simulink model "quy_dao_nghiem_so_2022"  (R2023b)
settings: Solver=VariableStepAuto  StartTime=0.0  StopTime=30000  MaxStep=20000.0  RelTol=1e-3
values from neighbouring files (symbols this model uses):
  A = 1    [doi_tuong.m]    (also in quy_dao_nghiem_so.m; tong_hop_truc_tiep.m)
  den = [1, a1, a2]    [quy_dao_nghiem_so.m]
  K1 = (alpha * l1_bar) / (2 * sqrt(delta_h))    [quy_dao_nghiem_so.m]
  K2 = (alpha * l2_bar) / (2 * sqrt(h2_bar))    [quy_dao_nghiem_so.m]
  K3 = alpha * sqrt(delta_h)    [quy_dao_nghiem_so.m]
  K4 = alpha * sqrt(h2_bar)    [quy_dao_nghiem_so.m]
libraries: simulink x2, slpidlib x2
settings Model: Creator=PC  LastModifiedBy=Moderator
settings SolverCC: ZeroCrossAlgorithm=Adaptive
settings DebuggingCC: IgnoredZcDiagnostic=none
settings RTWCC: GPUComputeCapability=5.0

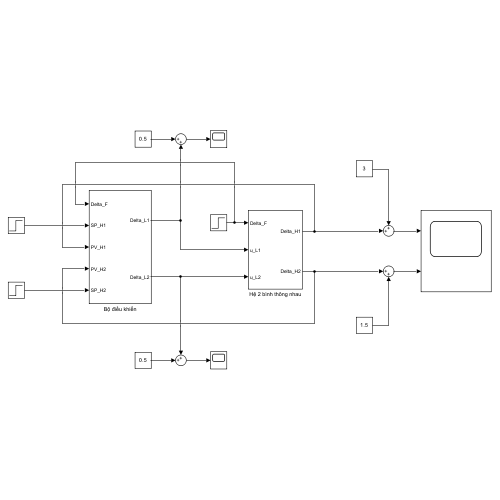
[thumbnail: Simulink's stored preview of the top-level diagram]
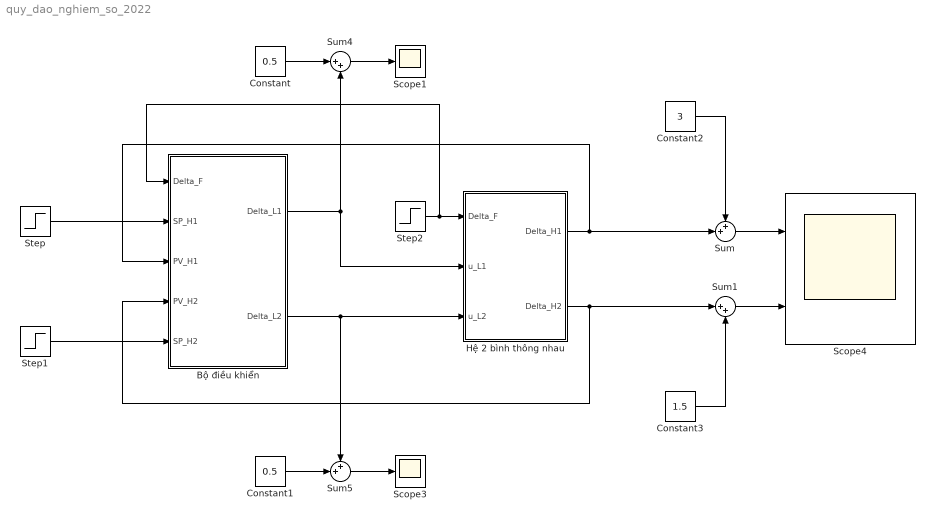
== system quy_dao_nghiem_so_2022 ==
  Bộ điều khiển : Subsystem
  Constant : Constant  Value=0.5
  Constant1 : Constant  Value=0.5
  Constant2 : Constant  Value=3
  Constant3 : Constant  Value=1.5
  Hệ 2 bình thông nhau : Subsystem
  Scope1 : Scope
  Scope3 : Scope
  Scope4 : Scope  NumInputPorts=2
  Step : Step  Time=20000  After=0.1  SampleTime=0
  Step1 : Step  Time=10000  After=0.1  SampleTime=0
  Step2 : Step  Time=10000  After=0.0002  SampleTime=0
  Sum : Sum  Inputs=++|
  Sum1 : Sum  Inputs=|++
  Sum4 : Sum  Inputs=|++
  Sum5 : Sum  Inputs=++|
  wires:
  Constant/1 -> Sum4/1
  Sum4/1 -> Scope1/1
  Sum5/1 -> Scope3/1
  Step2/1 -> Hệ 2 bình thông nhau/1(Delta_F), Bộ điều khiển/1(Delta_F)
  Constant1/1 -> Sum5/2
  Sum/1 -> Scope4/1
  Sum1/1 -> Scope4/2
  Constant2/1 -> Sum/1
  Constant3/1 -> Sum1/2
  Hệ 2 bình thông nhau/2(Delta_H2) -> Bộ điều khiển/4(PV_H2), Sum1/1
  Hệ 2 bình thông nhau/1(Delta_H1) -> Bộ điều khiển/3(PV_H1), Sum/2
  Bộ điều khiển/2(Delta_L2) -> Sum5/1, Hệ 2 bình thông nhau/3(u_L2)
  Bộ điều khiển/1(Delta_L1) -> Sum4/2, Hệ 2 bình thông nhau/2(u_L1)
  Step/1 -> Bộ điều khiển/2(SP_H1)
  Step1/1 -> Bộ điều khiển/5(SP_H2)

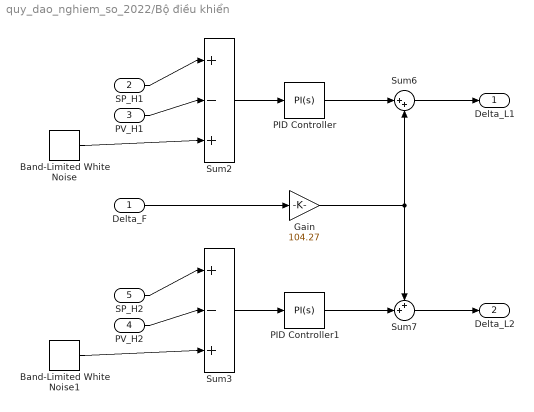
== system quy_dao_nghiem_so_2022/Bộ điều khiển ==
  Delta_F : Inport
  SP_H1 : Inport  Port=2
  PV_H1 : Inport  Port=3
  PV_H2 : Inport  Port=4
  SP_H2 : Inport  Port=5
  Band-Limited White Noise : simulink/Sources/Band-Limited White Noise  Cov=0.00001  Ts=0.1  seed=[23341]
  Band-Limited White Noise1 : simulink/Sources/Band-Limited White Noise  Cov=0.00001  Ts=0.1  seed=[23341]
  Gain : Gain  Gain=104.27
  PID Controller : slpidlib/PID Controller  Controller=PI  Form=Parallel  TimeDomain=Continuous-time  UseExternalTs=off  SampleTime=-1  IntegratorMethod=Forward Euler  FilterMethod=Forward Euler  ControllerParametersSource=internal  P=-1  I=-0.000195  UseKiTs=off  D=-653*0.55  N=50  UseFilter=on  TunerSelectOption=Transfer Function Based (PID Tuner App)  InitialConditionSource=internal  InitialConditionForIntegrator=0  InitialConditionForFilter=0  DifferentiatorICPrevScaledInput=0  ExternalReset=none  TrackingMode=off  Kt=1  LimitOutput=on  SatLimitsSource=internal  UpperSaturationLimit=0.5  LowerSaturationLimit=-0.5  LinearizeAsGain=on  AntiWindupMode=clamping  Kb=1  LimitIntegrator=off  UpperIntegratorSaturationLimit=inf  LowerIntegratorSaturationLimit=-inf  POutMin=[]  POutMax=[]  IOutMin=[]  IOutMax=[]  DOutMin=[]  DOutMax=[]  NOutMin=[]  NOutMax=[]  SumOutMin=[]  SumOutMax=[]  SaturationOutMin=[]  SaturationOutMax=[]  PParamMin=[]  PParamMax=[]  IParamMin=[]  IParamMax=[]  DParamMin=[]  DParamMax=[]  NParamMin=[]  NParamMax=[]  KbParamMin=[]  KbParamMax=[]  KtParamMin=[]  KtParamMax=[]  KbOutMin=[]  KbOutMax=[]  KtOutMin=[]  KtOutMax=[]  IntegratorOutMin=[]  IntegratorOutMax=[]  FilterOutMin=[]  FilterOutMax=[]  SumI1OutMin=[]  SumI1OutMax=[]  SumI2OutMin=[]  SumI2OutMax=[]  SumI3OutMin=[]  SumI3OutMax=[]  SumI4OutMin=[]  SumI4OutMax=[]  SumDOutMin=[]  SumDOutMax=[]  DifferentiatorOutMin=[]  DifferentiatorOutMax=[]  FilterDiffOutCoefMin=[]  FilterDiffOutCoefMax=[]  ReciprocalOutMin=[]  ReciprocalOutMax=[]  SumDenOutMin=[]  SumDenOutMax=[]  SumNumOutMin=[]  SumNumOutMax=[]  DivideOutMin=[]  DivideOutMax=[]  UdiffTsProdOutMin=[]  UdiffTsProdOutMax=[]  NTsProdOutMin=[]  NTsProdOutMax=[]  UintegralTsProdOutMin=[]  UintegralTsProdOutMax=[]  UngainTsProdOutMin=[]  UngainTsProdOutMax=[]  ClampingZeroOutDataTypeStr=Inherit: Inherit via back propagation  ClampingZeroOutMin=[]  ClampingZeroOutMax=[]  FilterDenConstantOutDataTypeStr=Inherit: Inherit via back propagation  FilterDenConstantOutMin=[]  FilterDenConstantOutMax=[]  PCopyOutDataTypeStr=Inherit: Inherit via back propagation  PCopyOutMin=[]  PCopyOutMax=[]  NCopyOutDataTypeStr=Inherit: Inherit via back propagation  NCopyOutMin=[]  NCopyOutMax=[]  IntegratorContinuousStateAttributes=''  IntegratorStateMustResolveToSignalObject=off  IntegratorRTWStateStorageClass=Auto  FilterContinuousStateAttributes=''  FilterStateMustResolveToSignalObject=off  FilterRTWStateStorageClass=Auto  ParallelPVariant=InternalParameters  IdealPVariant=Disabled  IVariant=InternalParameters  DVariant=Disabled  IntegratorVariant=Continuous  SatVariant=Enabled  AWVariant=ContClampingParallel  PCopyVariant=Disabled  TRVariant=Disabled  FdbkBlocksVariant=Forward  IdealPFdbkVariant=Disabled  SatFdbkVariant=Disabled  DerivativeFilterVariant=Disabled  NVariant=Disabled  NCopyVariant=Disabled_SignalSpec  FilterICVariant=Disabled  IntegratorICVariant=InternalICs  ExternalResetVariant=Disabled  TRSumVariant=Passthrough  SumFdbkVariant=Disabled  SumVariant=Sum_PI  TsampFilterVariant=InternalTs  TsampNgainVariant=Passthrough  TsampIntegralVariant=Disabled_SignalSpec  ExternalSaturationOutDataTypeStr=Inherit: Same as second input
  PID Controller1 : slpidlib/PID Controller  Controller=PI  Form=Parallel  TimeDomain=Continuous-time  UseExternalTs=off  SampleTime=-1  IntegratorMethod=Forward Euler  FilterMethod=Forward Euler  ControllerParametersSource=internal  P=-1  I=-0.000195  UseKiTs=off  D=-653*0.55  N=50  UseFilter=on  TunerSelectOption=Transfer Function Based (PID Tuner App)  InitialConditionSource=internal  InitialConditionForIntegrator=0  InitialConditionForFilter=0  DifferentiatorICPrevScaledInput=0  ExternalReset=none  TrackingMode=off  Kt=1  LimitOutput=on  SatLimitsSource=internal  UpperSaturationLimit=0.5  LowerSaturationLimit=-0.5  LinearizeAsGain=on  AntiWindupMode=clamping  Kb=1  LimitIntegrator=off  UpperIntegratorSaturationLimit=inf  LowerIntegratorSaturationLimit=-inf  POutMin=[]  POutMax=[]  IOutMin=[]  IOutMax=[]  DOutMin=[]  DOutMax=[]  NOutMin=[]  NOutMax=[]  SumOutMin=[]  SumOutMax=[]  SaturationOutMin=[]  SaturationOutMax=[]  PParamMin=[]  PParamMax=[]  IParamMin=[]  IParamMax=[]  DParamMin=[]  DParamMax=[]  NParamMin=[]  NParamMax=[]  KbParamMin=[]  KbParamMax=[]  KtParamMin=[]  KtParamMax=[]  KbOutMin=[]  KbOutMax=[]  KtOutMin=[]  KtOutMax=[]  IntegratorOutMin=[]  IntegratorOutMax=[]  FilterOutMin=[]  FilterOutMax=[]  SumI1OutMin=[]  SumI1OutMax=[]  SumI2OutMin=[]  SumI2OutMax=[]  SumI3OutMin=[]  SumI3OutMax=[]  SumI4OutMin=[]  SumI4OutMax=[]  SumDOutMin=[]  SumDOutMax=[]  DifferentiatorOutMin=[]  DifferentiatorOutMax=[]  FilterDiffOutCoefMin=[]  FilterDiffOutCoefMax=[]  ReciprocalOutMin=[]  ReciprocalOutMax=[]  SumDenOutMin=[]  SumDenOutMax=[]  SumNumOutMin=[]  SumNumOutMax=[]  DivideOutMin=[]  DivideOutMax=[]  UdiffTsProdOutMin=[]  UdiffTsProdOutMax=[]  NTsProdOutMin=[]  NTsProdOutMax=[]  UintegralTsProdOutMin=[]  UintegralTsProdOutMax=[]  UngainTsProdOutMin=[]  UngainTsProdOutMax=[]  ClampingZeroOutDataTypeStr=Inherit: Inherit via back propagation  ClampingZeroOutMin=[]  ClampingZeroOutMax=[]  FilterDenConstantOutDataTypeStr=Inherit: Inherit via back propagation  FilterDenConstantOutMin=[]  FilterDenConstantOutMax=[]  PCopyOutDataTypeStr=Inherit: Inherit via back propagation  PCopyOutMin=[]  PCopyOutMax=[]  NCopyOutDataTypeStr=Inherit: Inherit via back propagation  NCopyOutMin=[]  NCopyOutMax=[]  IntegratorContinuousStateAttributes=''  IntegratorStateMustResolveToSignalObject=off  IntegratorRTWStateStorageClass=Auto  FilterContinuousStateAttributes=''  FilterStateMustResolveToSignalObject=off  FilterRTWStateStorageClass=Auto  ParallelPVariant=InternalParameters  IdealPVariant=Disabled  IVariant=InternalParameters  DVariant=Disabled  IntegratorVariant=Continuous  SatVariant=Enabled  AWVariant=ContClampingParallel  PCopyVariant=Disabled  TRVariant=Disabled  FdbkBlocksVariant=Forward  IdealPFdbkVariant=Disabled  SatFdbkVariant=Disabled  DerivativeFilterVariant=Disabled  NVariant=Disabled  NCopyVariant=Disabled_SignalSpec  FilterICVariant=Disabled  IntegratorICVariant=InternalICs  ExternalResetVariant=Disabled  TRSumVariant=Passthrough  SumFdbkVariant=Disabled  SumVariant=Sum_PI  TsampFilterVariant=InternalTs  TsampNgainVariant=Passthrough  TsampIntegralVariant=Disabled_SignalSpec  ExternalSaturationOutDataTypeStr=Inherit: Same as second input
  Sum2 : Sum  Inputs=|+-+
  Sum3 : Sum  Inputs=|+-+
  Sum6 : Sum  Inputs=|++
  Sum7 : Sum  Inputs=++|
  Delta_L1 : Outport
  Delta_L2 : Outport  Port=2
  wires:
  PID Controller1/1 -> Sum7/2
  Sum2/1 -> PID Controller/1
  Gain/1 -> Sum6/2, Sum7/1
  SP_H1/1 -> Sum2/1
  PV_H2/1 -> Sum3/2
  Delta_F/1 -> Gain/1
  PID Controller/1 -> Sum6/1
  Sum3/1 -> PID Controller1/1
  Band-Limited White Noise/1 -> Sum2/3
  Band-Limited White Noise1/1 -> Sum3/3
  Sum6/1 -> Delta_L1/1
  SP_H2/1 -> Sum3/1
  PV_H1/1 -> Sum2/2
  Sum7/1 -> Delta_L2/1

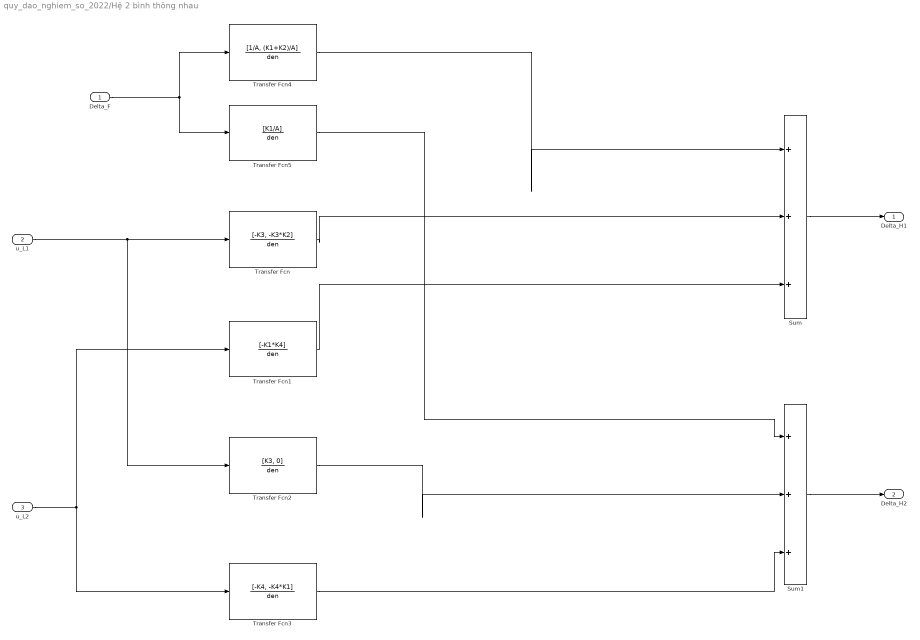
== system quy_dao_nghiem_so_2022/Hệ 2 bình thông nhau ==
  Delta_F : Inport
  u_L1 : Inport  Port=2
  u_L2 : Inport  Port=3
  Sum : Sum  Inputs=|+++
  Sum1 : Sum  Inputs=|+++
  Transfer Fcn : TransferFcn  Numerator=[-K3, -K3*K2]  Denominator=den
  Transfer Fcn1 : TransferFcn  Numerator=[-K1*K4]  Denominator=den
  Transfer Fcn2 : TransferFcn  Numerator=[K3, 0]  Denominator=den
  Transfer Fcn3 : TransferFcn  Numerator=[-K4, -K4*K1]  Denominator=den
  Transfer Fcn4 : TransferFcn  Numerator=[1/A, (K1+K2)/A]  Denominator=den
  Transfer Fcn5 : TransferFcn  Numerator=[K1/A]  Denominator=den
  Delta_H1 : Outport
  Delta_H2 : Outport  Port=2
  wires:
  Transfer Fcn5/1 -> Sum1/1
  u_L1/1 -> Transfer Fcn2/1, Transfer Fcn/1
  Transfer Fcn/1 -> Sum/2
  Transfer Fcn2/1 -> Sum1/2
  Transfer Fcn4/1 -> Sum/1
  Transfer Fcn3/1 -> Sum1/3
  Transfer Fcn1/1 -> Sum/3
  u_L2/1 -> Transfer Fcn1/1, Transfer Fcn3/1
  Delta_F/1 -> Transfer Fcn4/1, Transfer Fcn5/1
  Sum/1 -> Delta_H1/1
  Sum1/1 -> Delta_H2/1
